simulink model "q1cd"  (R2025b)
settings: Solver=ode45  StartTime=0.0  StopTime=30  RelTol=1e-3
settings Model: Creator=z.yin  LastModifiedBy=z.yin

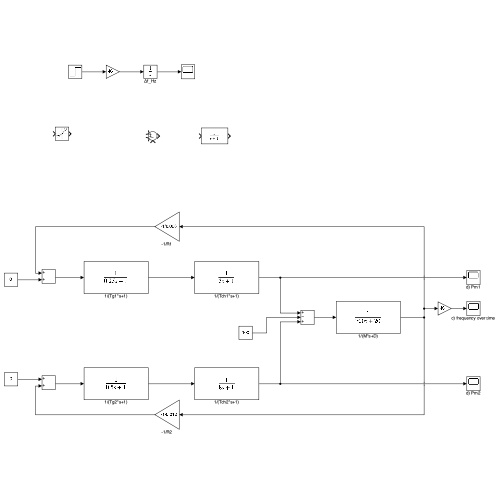
[thumbnail: Simulink's stored preview of the top-level diagram]
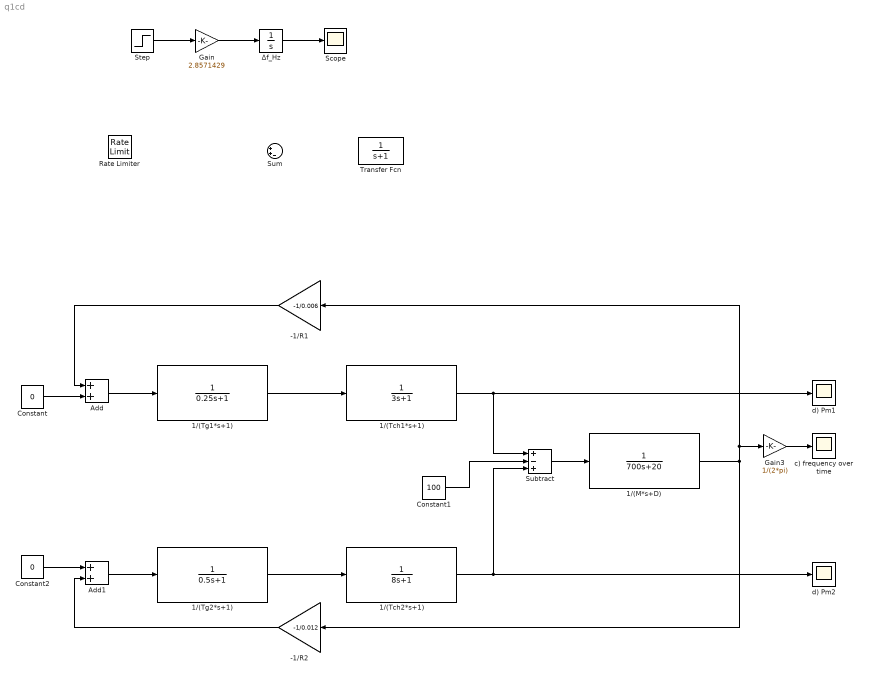
== system q1cd ==
  -1/R1 : Gain  Gain=-1/0.006
  -1/R2 : Gain  Gain=-1/0.012
  1/(M*s+D) : TransferFcn  Denominator=[700 20]
  1/(Tch1*s+1) : TransferFcn  Denominator=[3 1]
  1/(Tch2*s+1) : TransferFcn  Denominator=[8 1]
  1/(Tg1*s+1) : TransferFcn  Denominator=[0.25 1]
  1/(Tg2*s+1) : TransferFcn  Denominator=[0.5 1]
  Add : Sum
  Add1 : Sum
  Constant : Constant  Value=0
  Constant1 : Constant  Value=100
  Constant2 : Constant  Value=0
  Gain : Gain  Gain=2.8571429
  Gain3 : Gain  Gain=1/(2*pi)
  Rate Limiter : RateLimiter  SampleTimeMode=inherited
  Scope : Scope
  Step : Step  Time=0  After=0.05  SampleTime=0
  Subtract : Sum  Inputs=+-+
  Sum : Sum  Inputs=|++-
  Transfer Fcn : TransferFcn  Denominator=[1 1]
  c) frequency over time : Scope
      settings: ActiveDisplayYMinimum=-0.1009377694690614  ActiveDisplayYMaximum=0.011215307718784599  DataLoggingVariableName=deltaF
  d) Pm1 : Scope
      settings: ActiveDisplayYMinimum=-13.79191550661649  ActiveDisplayYMaximum=97.653496118051692  DataLoggingVariableName=Pm1
  d) Pm2 : Scope
      settings: ActiveDisplayYMinimum=-3.9741691062345192  ActiveDisplayYMaximum=35.767521956110684  DataLoggingVariableName=Pm2
  Δf_Hz : Integrator
  wires:
  Step/1 -> Gain/1
  Gain/1 -> Δf_Hz/1
  Δf_Hz/1 -> Scope/1
  1/(Tg2*s+1)/1 -> 1/(Tch2*s+1)/1
  1/(Tch2*s+1)/1 -> d) Pm2/1, Subtract/3
  1/(Tg1*s+1)/1 -> 1/(Tch1*s+1)/1
  1/(M*s+D)/1 -> -1/R2/1, Gain3/1, -1/R1/1
  Constant1/1 -> Subtract/2
  Add1/1 -> 1/(Tg2*s+1)/1
  1/(Tch1*s+1)/1 -> d) Pm1/1, Subtract/1
  Constant2/1 -> Add1/1
  -1/R2/1 -> Add1/2
  Gain3/1 -> c) frequency over time/1
  Subtract/1 -> 1/(M*s+D)/1
  -1/R1/1 -> Add/1
  Add/1 -> 1/(Tg1*s+1)/1
  Constant/1 -> Add/2
